simulink model "AV9_4"  (R2018a)
settings: Solver=VariableStepAuto  StartTime=0.0  StopTime=100  RelTol=1e-3
values from neighbouring files (symbols this model uses):
  q0 = -1.1901    [AV10_ZADACHA1.m]    (also in AV9_PRIMER2_VREDNOSTI.m = -62.3782; AV9_PRIMER4.m = 1.9573; AV9_PRIMER5.m = 1.8649; AV_10_PRIMER1.m = 1.512)
  q1 = 0.8945    [AV10_ZADACHA1.m]    (also in AV9_PRIMER2_VREDNOSTI.m = 122.0694; AV9_PRIMER4.m = -1.6594; AV9_PRIMER5.m = -1.8649; AV_10_PRIMER1.m = -1.423)
  q2 = -0.2805    [AV10_ZADACHA1.m]    (also in AV9_PRIMER2_VREDNOSTI.m = -59.9743; AV9_PRIMER4.m = 0.6675; AV9_PRIMER5.m = 0.2403; AV_10_PRIMER1.m = 0.44)
  T = 160    [AV10_ZADACHA1.m]    (also in AV9_PRIMER4.m = 16; AV9_PRIMER5.m = 4; AV_10_PRIMER1.m = 8)
settings Model: Creator=DD  LastModifiedBy=DD

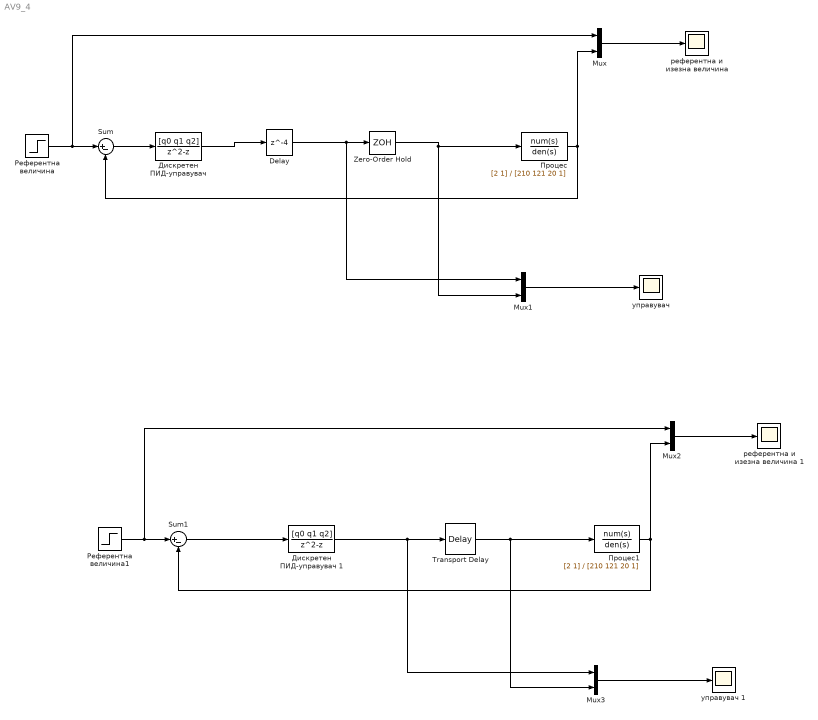
== system AV9_4 ==
  Delay : Delay  DelayLength=4  InitialCondition=0
  Mux{,1..3} (4 alike) : Mux  Inputs=2
  Sum : Sum  Inputs=|+-
  Sum1 : Sum  Inputs=|+-
  Transport Delay : TransportDelay  DelayTime=4
  Zero-Order Hold : ZeroOrderHold  SampleTime=T
  "Дискретен ПИД-управувач " : DiscreteTransferFcn  Numerator=[q0 q1 q2]  Denominator=[1 -1 0 ]  SampleTime=T
  Дискретен ПИД-управувач 1 : DiscreteTransferFcn  Numerator=[q0 q1 q2]  Denominator=[1 -1 0 ]  SampleTime=T
  Процес : TransferFcn  Numerator=[2 1]  Denominator=[210 121 20 1]
  Процес1 : TransferFcn  Numerator=[2 1]  Denominator=[210 121 20 1]
  Референтна величина : Step  SampleTime=0
  Референтна величина1 : Step  SampleTime=0
  "референтна и изезна величина " : Scope
  референтна и изезна величина 1 : Scope
  "управувач " : Scope
  управувач 1 : Scope
  wires:
  "Дискретен ПИД-управувач "/1 -> Delay/1
  Zero-Order Hold/1 -> Mux1/2, Процес/1
  Sum/1 -> "Дискретен ПИД-управувач "/1
  Референтна величина/1 -> Mux/1, Sum/1
  Процес/1 -> Mux/2, Sum/2
  Mux/1 -> "референтна и изезна величина "/1
  Mux1/1 -> "управувач "/1
  Mux2/1 -> референтна и изезна величина 1/1
  Transport Delay/1 -> Mux3/2, Процес1/1
  Дискретен ПИД-управувач 1/1 -> Transport Delay/1, Mux3/1
  Референтна величина1/1 -> Mux2/1, Sum1/1
  Процес1/1 -> Mux2/2, Sum1/2
  Sum1/1 -> Дискретен ПИД-управувач 1/1
  Mux3/1 -> управувач 1/1
  Delay/1 -> Mux1/1, Zero-Order Hold/1
